simulink model "CubeQuat"  (R2016a)
settings: Solver=ode45  StartTime=0.0  StopTime=t_stop  RelTol=rel_tol
values from neighbouring files (symbols this model uses):
  adr1 = ADRblockGen(wo1,I(1,1),3)    [CubeQuat_setup.m]
  adr2 = ADRblockGen(wo2,I(2,2),3)    [CubeQuat_setup.m]    (also in WBC_setup.m = ADRblockGen(w2,m,3))
  adr3 = ADRblockGen(wo3,I(3,3),3)    [CubeQuat_setup.m]
  control_selec = 2    [CubeQuat_setup.m]
  distrej1 = 1    [CubeQuat_setup.m]
  distrej2 = 1    [CubeQuat_setup.m]
  distrej3 = 1    [CubeQuat_setup.m]
  euler_init = [0;0;0]    [CubeQuat_setup.m]
  I = diag(I_mom) + [0 I_prd(1) I_prd(2); I_prd(1) 0 I_prd(3); I_prd(2) I_prd(3) 0]    [CubeQuat_setup.m]    (also in CubeSatModel.m = reshape(I,3,3); CubeSatSfun.m = block.DialogPrm(2).Data; CubeSimSetUp.m = diag([Ixx;Iyy;Izz]); Satellite_Setup.m = diag([Ixx;Iyy;Izz]))
  in_cond_selec = 1    [CubeQuat_setup.m]
  k1 = 10    [CubeQuat_setup.m]    (also in WS_20_09_2017.mat = 5e-08; WS_25_09_2017.mat = 5e-08)
  k2 = 10    [CubeQuat_setup.m]    (also in WBC_setup.m = 5e-09; WS_20_09_2017.mat = 5e-09; WS_25_09_2017.mat = 5e-09; WS_29_09_2017.mat = 1.56433333333e-08)
  k3 = 10    [CubeQuat_setup.m]
  kd = 6e-4    (= 0.0006)    [Control_mission_def.m]    (also in CubeQuat_setup.m = 2*sqrt(I(1,1))*sqrt(kp); CubeSimSetUp.m; Example__simulaltion.m; Example_simulaltion.m)
  kp = 5e-9    (= 5e-09)    [Control_mission_def.m]    (also in CubeQuat_setup.m = 40; CubeSimSetUp.m; Example__simulaltion.m; Example_simulaltion.m)
  M = zeros(3,1)    [CubeQuat_setup.m]
  mass = 15    [CubeQuat_setup.m]    (also in CubeSimSetUp.m = 2.6; Satellite_Setup.m = 2.6; Satellite_Setup_Sun_Pointing.m = 2.6; Satellite_setup_ZenithPointing.m = 2.6)
  omega_0 = [30;30;30]*(1/sqrt(3))*(pi/180)    [CubeQuat_setup.m]
  omega_orbit = [0;-7.67/(401.1+6371);0]    [CubeQuat_setup.m]    (also in CubeSatModel.m = inputs(28:30); CubeSatSfun.m = block.DialogPrm(3).Data; CubeSimSetUp.m; Satellite_Setup.m)
  x = inputs(1:18)    [CubeSatModel.m]
  x_0 = [0,0,0,1,0,0,0]    [CubeQuat_setup.m]    (also in CubeSimSetUp.m = [wb_bi_init;qb_o_init;qb_i_init;qo_i_init;long_init;lat_init; Example__simulaltion.m = transpose([wb_bi_init,qb_i_init]); Example_simulaltion.m = transpose([wb_bi_init,qb_i_init]); Satellite_Setup.m = transpose([wb_bi_init,qb_i_init]))
undefined symbols (not defined in the file or in its folder): rotationalDynamics
libraries: cstblocks x24, aerolibtransform2 x3
settings Model: Creator=Daire  LastModifiedBy=vicubso
settings DataIOCC: LimitDataPoints=on  SaveFormat=Array
settings DebuggingCC: SolverPrmCheckMsg=warning
settings HardwareCC: ProdBitPerPointer=32  ProdLargestAtomicFloat=None  ProdIntDivRoundTo=Undefined  ProdEndianess=Unspecified  ProdWordSize=32  ProdHWDeviceType=32-bit Generic
settings ModelReferenceCC: PropagateSignalLabelsOutOfModel=off
settings ConfigComp: CovModelRefEnable=Off  CovSFcnEnable=off
settings ConfigurationSet: Description=SimMechanics 2G

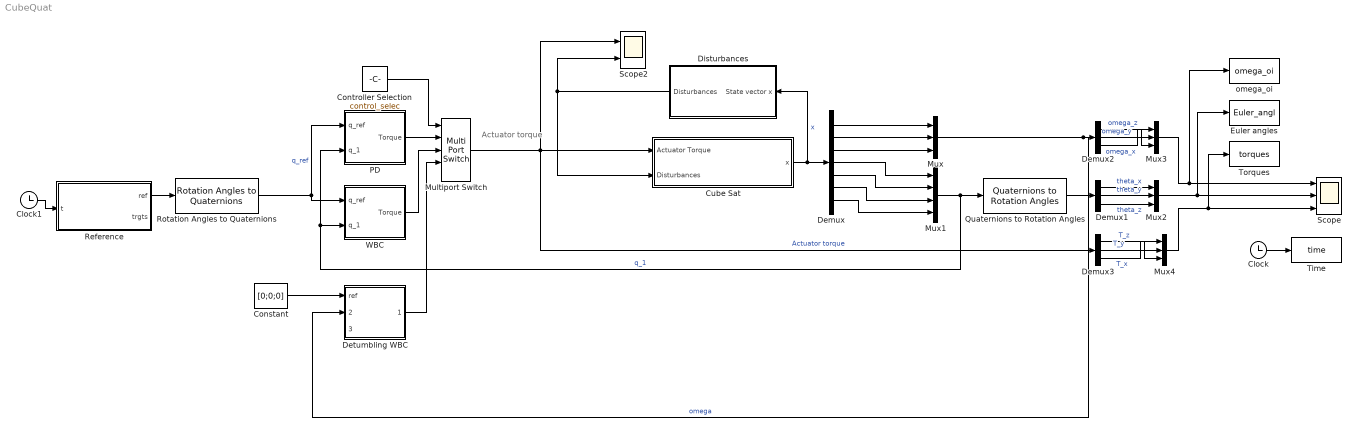
== system CubeQuat ==
  note: Actuator torque
  Clock : Clock
  Clock1 : Clock
  Constant : Constant  Value=[0;0;0]
  Controller Selection : Constant  Value=control_selec
  Cube Sat : Subsystem
  Demux : Demux  Outputs=7
  Demux1 : Demux  Outputs=3
  Demux2 : Demux  Outputs=3
  Demux3 : Demux  Outputs=3
  Detumbling WBC : Subsystem
  Disturbances : Subsystem
  Euler angles : ToWorkspace  VariableName=Euler_angl  SampleTime=-1
  Multiport Switch : MultiPortSwitch  Inputs=4
  Mux{,2..4} (4 alike) : Mux  Inputs=3
  Mux1 : Mux
  PD : Subsystem
  Quaternions to Rotation Angles : aerolibtransform2/Quaternions to Rotation Angles  rotationOrder=ZYX
  Reference : MATLAB Function  TreatAsAtomicUnit=on
  Rotation Angles to Quaternions : aerolibtransform2/Rotation Angles to Quaternions  rotationOrder=ZYX
  Scope : Scope  NumInputPorts=3
  Scope2 : Scope  NumInputPorts=2
  Time : ToWorkspace  VariableName=time  SampleTime=-1
  Torques : ToWorkspace  VariableName=torques  SampleTime=-1
  WBC : Subsystem
  omega_oi : ToWorkspace  VariableName=omega_oi  SampleTime=-1
  wires:
  Demux/1 -> Mux/1
  Demux/2 -> Mux/2
  Demux/3 -> Mux/3
  Demux/4 -> Mux1/1
  Demux/5 -> Mux1/2
  Demux/6 -> Mux1/3
  Demux/7 -> Mux1/4
  Mux1/1 -> Quaternions to Rotation Angles/1, PD/2(q_1), WBC/2(q_1)  "q_1"
  Quaternions to Rotation Angles/1 -> Demux1/1
  Rotation Angles to Quaternions/1 -> PD/1(q_ref), WBC/1(q_ref)  "q_ref"
  Demux1/1 -> Mux2/1  "theta_x"
  Demux1/2 -> Mux2/2  "theta_y"
  Demux1/3 -> Mux2/3  "theta_z"
  Mux2/1 -> Euler angles/1, Scope/2
  Mux/1 -> Detumbling WBC/2(omega), Demux2/1  "omega"
  Demux2/1 -> Mux3/3  "omega_z"
  Demux2/2 -> Mux3/2  "omega_y"
  Demux2/3 -> Mux3/1  "omega_x"
  Mux3/1 -> Scope/1, omega_oi/1
  Cube Sat/1(x) -> Disturbances/1(State vector x), Demux/1  "x"
  Multiport Switch/1 -> Scope2/1, Demux3/1, Cube Sat/1(Actuator Torque)  "Actuator torque"
  PD/1(Torque) -> Multiport Switch/2
  Mux4/1 -> Torques/1, Scope/3
  Demux3/1 -> Mux4/3  "T_z"
  Demux3/3 -> Mux4/1  "T_x"
  Demux3/2 -> Mux4/2  "T_y"
  Controller Selection/1 -> Multiport Switch/1
  Clock/1 -> Time/1
  WBC/1(Torque) -> Multiport Switch/3
  Disturbances/1(Disturbances) -> Cube Sat/2(Disturbances), Scope2/2
  Constant/1 -> Detumbling WBC/1(ref)
  Detumbling WBC/1(Torque) -> Multiport Switch/4
  Clock1/1 -> Reference/1(t)
  Reference/1(ref) -> Rotation Angles to Quaternions/1

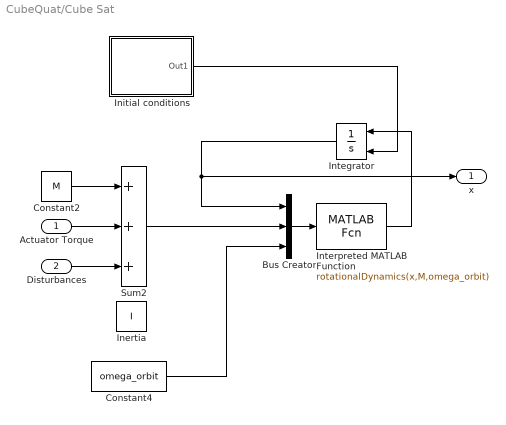
== system CubeQuat/Cube Sat ==
  Actuator Torque : Inport
  Disturbances : Inport  Port=2
  Bus Creator : BusCreator  Inputs=3
  Constant2 : Constant  Value=M
  Constant4 : Constant  Value=omega_orbit
  Inertia : Constant  Value=I
  Initial conditions : Subsystem
  Integrator : Integrator  InitialConditionSource=external
  Interpreted MATLAB Function : MATLABFcn  MATLABFcn=rotationalDynamics(x,M,omega_orbit)  OutputDimensions=1
  Sum2 : Sum  Inputs=+++
  x : Outport
  wires:
  Sum2/1 -> Bus Creator/2
  Integrator/1 -> Bus Creator/1, x/1
  Constant2/1 -> Sum2/1
  Interpreted MATLAB Function/1 -> Integrator/1
  Actuator Torque/1 -> Sum2/2
  Initial conditions/1(Out1) -> Integrator/2
  Constant4/1 -> Bus Creator/3
  Disturbances/1 -> Sum2/3
  Bus Creator/1 -> Interpreted MATLAB Function/1

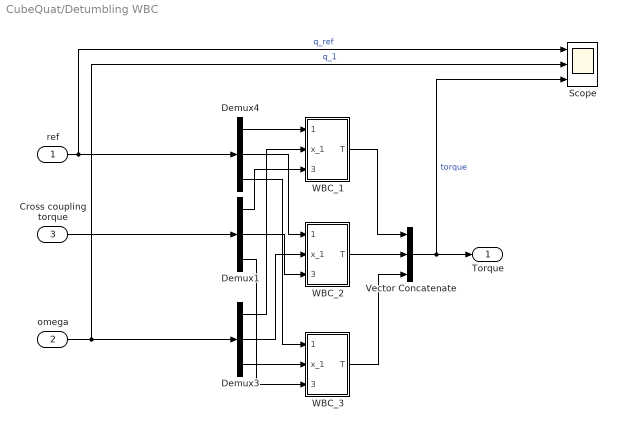
== system CubeQuat/Detumbling WBC ==
  ref : Inport
  omega : Inport  Port=2
  Cross coupling torque : Inport  Port=3
  Demux1 : Demux  Outputs=3
  Demux3 : Demux  Outputs=3
  Demux4 : Demux  Outputs=3
  Scope : Scope  NumInputPorts=3
  Vector Concatenate : Concatenate  NumInputs=3
  WBC_1 : Subsystem
  WBC_2 : Subsystem
  WBC_3 : Subsystem
  Torque : Outport
  wires:
  Demux1/3 -> WBC_3/3(Cross coupling torque)
  Demux1/2 -> WBC_2/3(Cross coupling torque)
  Demux1/1 -> WBC_1/3(Cross coupling torque)
  Cross coupling torque/1 -> Demux1/1
  WBC_1/1(T) -> Vector Concatenate/1
  Demux3/1 -> WBC_1/2(x_1)
  Demux3/2 -> WBC_2/2(x_1)
  Demux4/2 -> WBC_2/1(x_0_ref)
  ref/1 -> Demux4/1, Scope/1  "q_ref"
  WBC_3/1(T) -> Vector Concatenate/3
  Vector Concatenate/1 -> Scope/3, Torque/1  "torque"
  WBC_2/1(T) -> Vector Concatenate/2
  Demux4/3 -> WBC_3/1(x_0_ref)
  Demux4/1 -> WBC_1/1(x_0_ref)
  omega/1 -> Demux3/1, Scope/2  "q_1"
  Demux3/3 -> WBC_3/2(x_1)

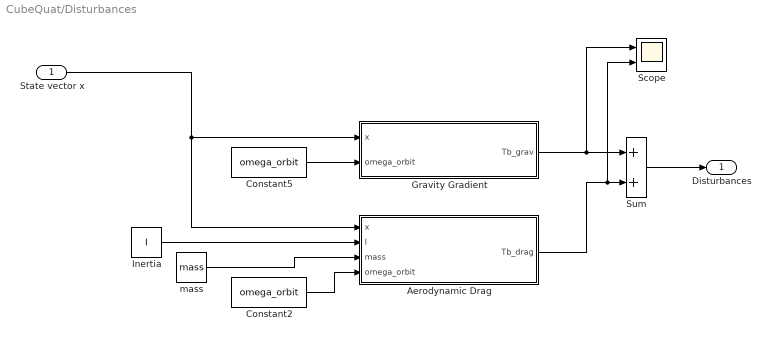
== system CubeQuat/Disturbances ==
  State vector x : Inport
  Aerodynamic Drag : MATLAB Function  TreatAsAtomicUnit=on
  Constant2 : Constant  Value=omega_orbit
  Constant5 : Constant  Value=omega_orbit
  Gravity Gradient : MATLAB Function  TreatAsAtomicUnit=on
  Inertia : Constant  Value=I
  Scope : Scope  NumInputPorts=2
  Sum : Sum
  mass : Constant  Value=mass
  Disturbances : Outport
  wires:
  Aerodynamic Drag/1(Tb_drag) -> Scope/2, Sum/2
  mass/1 -> Aerodynamic Drag/3(mass)
  Constant5/1 -> Gravity Gradient/2(omega_orbit)
  Constant2/1 -> Aerodynamic Drag/4(omega_orbit)
  Inertia/1 -> Aerodynamic Drag/2(I)
  State vector x/1 -> Gravity Gradient/1(x), Aerodynamic Drag/1(x)
  Sum/1 -> Disturbances/1
  Gravity Gradient/1(Tb_grav) -> Scope/1, Sum/1

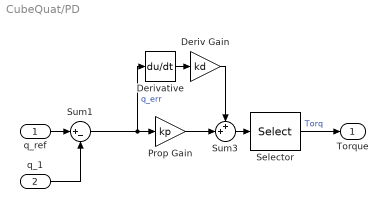
== system CubeQuat/PD ==
  q_ref : Inport
  q_1 : Inport  Port=2
  Deriv Gain : Gain  Gain=kd
  Derivative : Derivative
  Prop Gain : Gain  Gain=kp
  Selector : Selector  InputPortWidth=4  IndexOptions=Index vector (dialog)  Indices=[2,3,4]  OutputSizes=1
  Sum1 : Sum  Inputs=|+-
  Sum3 : Sum  Inputs=++|
  Torque : Outport
  wires:
  Selector/1 -> Torque/1  "Torq"
  Deriv Gain/1 -> Sum3/1
  Derivative/1 -> Deriv Gain/1
  Prop Gain/1 -> Sum3/2
  Sum1/1 -> Prop Gain/1, Derivative/1  "q_err"
  q_1/1 -> Sum1/2
  q_ref/1 -> Sum1/1
  Sum3/1 -> Selector/1

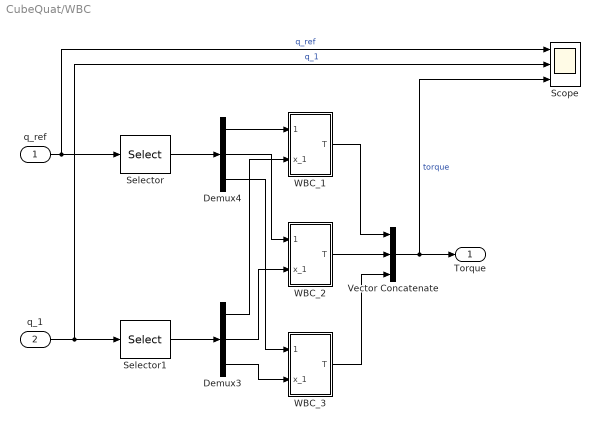
== system CubeQuat/WBC ==
  q_ref : Inport
  q_1 : Inport  Port=2
  Demux3 : Demux  Outputs=3
  Demux4 : Demux  Outputs=3
  Scope : Scope  NumInputPorts=3
  Selector : Selector  InputPortWidth=4  IndexOptions=Index vector (dialog)  Indices=[2,3,4]  OutputSizes=1
  Selector1 : Selector  InputPortWidth=4  IndexOptions=Index vector (dialog)  Indices=[2,3,4]  OutputSizes=1
  Vector Concatenate : Concatenate  NumInputs=3
  WBC_1 : Subsystem
  WBC_2 : Subsystem
  WBC_3 : Subsystem
  Torque : Outport
  wires:
  Demux3/3 -> WBC_3/2(x_1)
  q_1/1 -> Scope/2, Selector1/1  "q_1"
  Demux4/1 -> WBC_1/1(x_0_ref)
  Demux4/3 -> WBC_3/1(x_0_ref)
  WBC_2/1(T) -> Vector Concatenate/2
  Vector Concatenate/1 -> Torque/1, Scope/3  "torque"
  WBC_3/1(T) -> Vector Concatenate/3
  q_ref/1 -> Selector/1, Scope/1  "q_ref"
  Selector/1 -> Demux4/1
  Demux4/2 -> WBC_2/1(x_0_ref)
  Selector1/1 -> Demux3/1
  Demux3/2 -> WBC_2/2(x_1)
  Demux3/1 -> WBC_1/2(x_1)
  WBC_1/1(T) -> Vector Concatenate/1

== system CubeQuat/Cube Sat/Initial conditions ==
  Initial Cond. Selector : Constant  Value=in_cond_selec
  Initial Conditions : Constant  Value=x_0
  Initial Conditions1 : Constant  Value=omega_0
  Initial Conditions2 : Constant  Value=euler_init
  Mux : Mux  Inputs=2
  Rotation Angles to Quaternions : aerolibtransform2/Rotation Angles to Quaternions  rotationOrder=ZYX
  Switch : Switch  Criteria=u2 ~= 0
  Out1 : Outport
  wires:
  Initial Conditions/1 -> Switch/1
  Rotation Angles to Quaternions/1 -> Mux/2
  Switch/1 -> Out1/1
  Mux/1 -> Switch/3
  Initial Conditions1/1 -> Mux/1
  Initial Conditions2/1 -> Rotation Angles to Quaternions/1
  Initial Cond. Selector/1 -> Switch/2

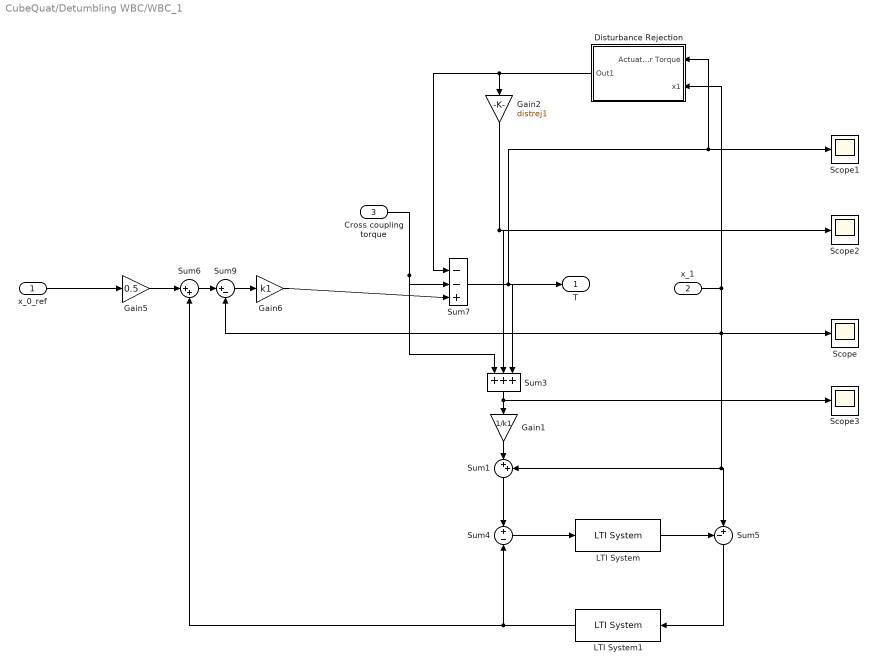
== system CubeQuat/Detumbling WBC/WBC_1 ==
  x_0_ref : Inport
  x_1 : Inport  Port=2
  Cross coupling torque : Inport  Port=3
  Disturbance Rejection : Subsystem
  Gain1 : Gain  Gain=1/k1
  Gain2 : Gain  Gain=distrej1
  Gain5 : Gain  Gain=0.5
  Gain6 : Gain  Gain=k1
  LTI System : cstblocks/LTI System  sys=G1  IC=[]
  LTI System1 : cstblocks/LTI System  sys=G1  IC=[]
  Scope{,1..3} (4 alike) : Scope
  Sum1 : Sum  Inputs=|++
  Sum3 : Sum  Inputs=+++|
  Sum4 : Sum  Inputs=+|-
  Sum5 : Sum  Inputs=-+|
  Sum6 : Sum  Inputs=|++
  Sum7 : Sum  Inputs=--+|
  Sum9 : Sum  Inputs=|+-
  T : Outport
  wires:
  Cross coupling torque/1 -> Sum7/2, Sum3/1
  Disturbance Rejection/1(Out1) -> Gain2/1, Sum7/1
  x_1/1 -> Disturbance Rejection/2(x1), Sum9/2, Scope/1, Sum5/2, Sum1/2
  Gain1/1 -> Sum1/1
  LTI System1/1 -> Sum6/2, Sum4/2
  Gain2/1 -> Scope2/1, Sum3/2
  Gain6/1 -> Sum7/3
  Sum3/1 -> Gain1/1, Scope3/1
  Sum6/1 -> Sum9/1
  x_0_ref/1 -> Gain5/1
  Sum9/1 -> Gain6/1
  Sum7/1 -> T/1, Sum3/3, Disturbance Rejection/1(Actuator Torque), Scope1/1
  Gain5/1 -> Sum6/1
  Sum4/1 -> LTI System/1
  LTI System/1 -> Sum5/1
  Sum5/1 -> LTI System1/1
  Sum1/1 -> Sum4/1

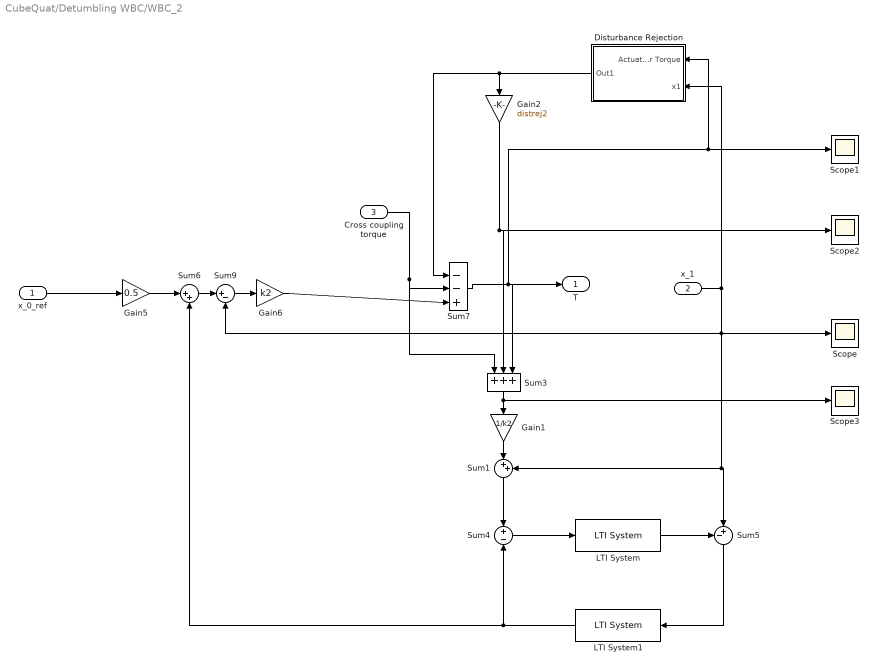
== system CubeQuat/Detumbling WBC/WBC_2 ==
  x_0_ref : Inport
  x_1 : Inport  Port=2
  Cross coupling torque : Inport  Port=3
  Disturbance Rejection : Subsystem
  Gain1 : Gain  Gain=1/k2
  Gain2 : Gain  Gain=distrej2
  Gain5 : Gain  Gain=0.5
  Gain6 : Gain  Gain=k2
  LTI System : cstblocks/LTI System  sys=G2  IC=[]
  LTI System1 : cstblocks/LTI System  sys=G2  IC=[]
  Scope{,1..3} (4 alike) : Scope
  Sum1 : Sum  Inputs=|++
  Sum3 : Sum  Inputs=+++|
  Sum4 : Sum  Inputs=+|-
  Sum5 : Sum  Inputs=-+|
  Sum6 : Sum  Inputs=|++
  Sum7 : Sum  Inputs=--+|
  Sum9 : Sum  Inputs=|+-
  T : Outport
  wires:
  Cross coupling torque/1 -> Sum3/1, Sum7/2
  Disturbance Rejection/1(Out1) -> Gain2/1, Sum7/1
  x_1/1 -> Disturbance Rejection/2(x1), Sum9/2, Scope/1, Sum5/2, Sum1/2
  Gain1/1 -> Sum1/1
  LTI System1/1 -> Sum6/2, Sum4/2
  Gain2/1 -> Scope2/1, Sum3/2
  Gain6/1 -> Sum7/3
  Sum3/1 -> Gain1/1, Scope3/1
  Sum6/1 -> Sum9/1
  x_0_ref/1 -> Gain5/1
  Sum9/1 -> Gain6/1
  Sum7/1 -> T/1, Sum3/3, Disturbance Rejection/1(Actuator Torque), Scope1/1
  Gain5/1 -> Sum6/1
  Sum4/1 -> LTI System/1
  LTI System/1 -> Sum5/1
  Sum5/1 -> LTI System1/1
  Sum1/1 -> Sum4/1

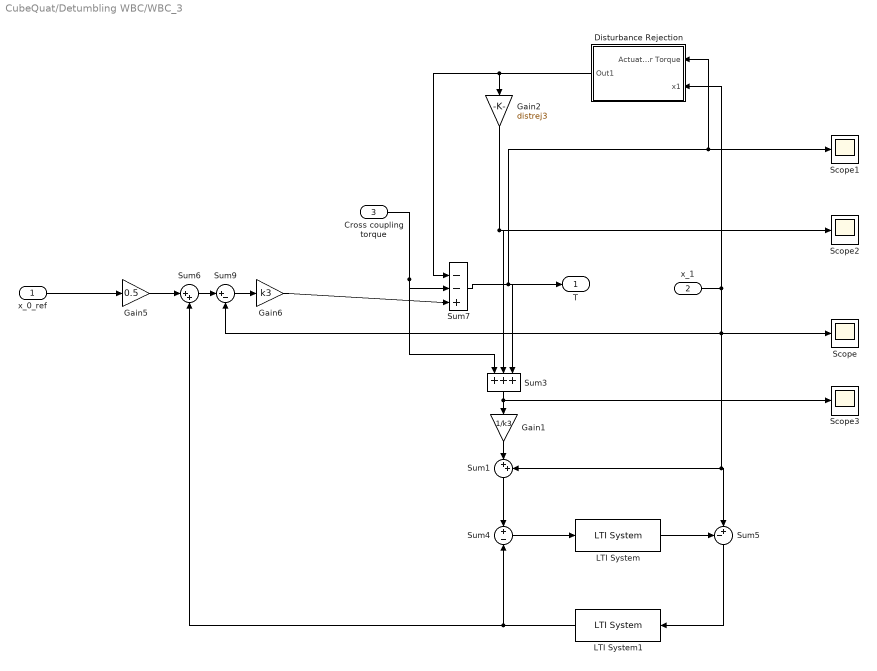
== system CubeQuat/Detumbling WBC/WBC_3 ==
  x_0_ref : Inport
  x_1 : Inport  Port=2
  Cross coupling torque : Inport  Port=3
  Disturbance Rejection : Subsystem
  Gain1 : Gain  Gain=1/k3
  Gain2 : Gain  Gain=distrej3
  Gain5 : Gain  Gain=0.5
  Gain6 : Gain  Gain=k3
  LTI System : cstblocks/LTI System  sys=G3  IC=[]
  LTI System1 : cstblocks/LTI System  sys=G3  IC=[]
  Scope{,1..3} (4 alike) : Scope
  Sum1 : Sum  Inputs=|++
  Sum3 : Sum  Inputs=+++|
  Sum4 : Sum  Inputs=+|-
  Sum5 : Sum  Inputs=-+|
  Sum6 : Sum  Inputs=|++
  Sum7 : Sum  Inputs=--+|
  Sum9 : Sum  Inputs=|+-
  T : Outport
  wires:
  Cross coupling torque/1 -> Sum3/1, Sum7/2
  Disturbance Rejection/1(Out1) -> Gain2/1, Sum7/1
  x_1/1 -> Disturbance Rejection/2(x1), Sum9/2, Scope/1, Sum5/2, Sum1/2
  Gain1/1 -> Sum1/1
  LTI System1/1 -> Sum6/2, Sum4/2
  Gain2/1 -> Scope2/1, Sum3/2
  Gain6/1 -> Sum7/3
  Sum3/1 -> Gain1/1, Scope3/1
  Sum6/1 -> Sum9/1
  x_0_ref/1 -> Gain5/1
  Sum9/1 -> Gain6/1
  Sum7/1 -> T/1, Sum3/3, Disturbance Rejection/1(Actuator Torque), Scope1/1
  Gain5/1 -> Sum6/1
  Sum4/1 -> LTI System/1
  LTI System/1 -> Sum5/1
  Sum5/1 -> LTI System1/1
  Sum1/1 -> Sum4/1

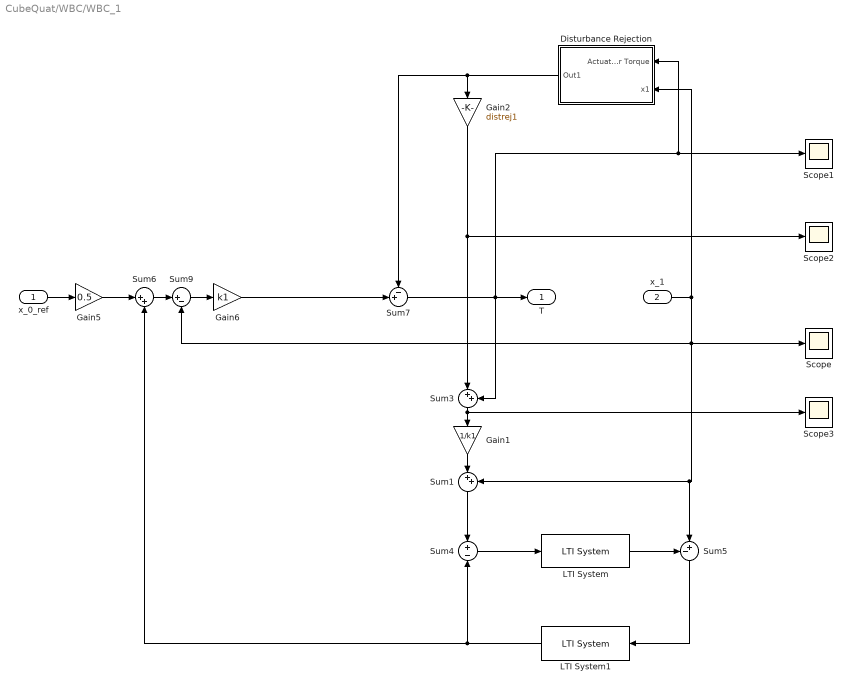
== system CubeQuat/WBC/WBC_1 ==
  x_0_ref : Inport
  x_1 : Inport  Port=2
  Disturbance Rejection : Subsystem
  Gain1 : Gain  Gain=1/k1
  Gain2 : Gain  Gain=distrej1
  Gain5 : Gain  Gain=0.5
  Gain6 : Gain  Gain=k1
  LTI System : cstblocks/LTI System  sys=G1  IC=[]
  LTI System1 : cstblocks/LTI System  sys=G1  IC=[]
  Scope{,1..3} (4 alike) : Scope
  Sum1 : Sum  Inputs=|++
  Sum3 : Sum  Inputs=|++
  Sum4 : Sum  Inputs=+|-
  Sum5 : Sum  Inputs=-+|
  Sum6 : Sum  Inputs=|++
  Sum7 : Sum  Inputs=-+|
  Sum9 : Sum  Inputs=|+-
  T : Outport
  wires:
  Sum1/1 -> Sum4/1
  Sum5/1 -> LTI System1/1
  LTI System/1 -> Sum5/1
  Sum4/1 -> LTI System/1
  Gain5/1 -> Sum6/1
  Sum7/1 -> Scope1/1, Disturbance Rejection/1(Actuator Torque), Sum3/2, T/1
  Sum9/1 -> Gain6/1
  x_0_ref/1 -> Gain5/1
  Sum6/1 -> Sum9/1
  Sum3/1 -> Scope3/1, Gain1/1
  Gain6/1 -> Sum7/2
  Gain2/1 -> Sum3/1, Scope2/1
  LTI System1/1 -> Sum4/2, Sum6/2
  Gain1/1 -> Sum1/1
  x_1/1 -> Sum1/2, Sum5/2, Scope/1, Sum9/2, Disturbance Rejection/2(x1)
  Disturbance Rejection/1(Out1) -> Sum7/1, Gain2/1

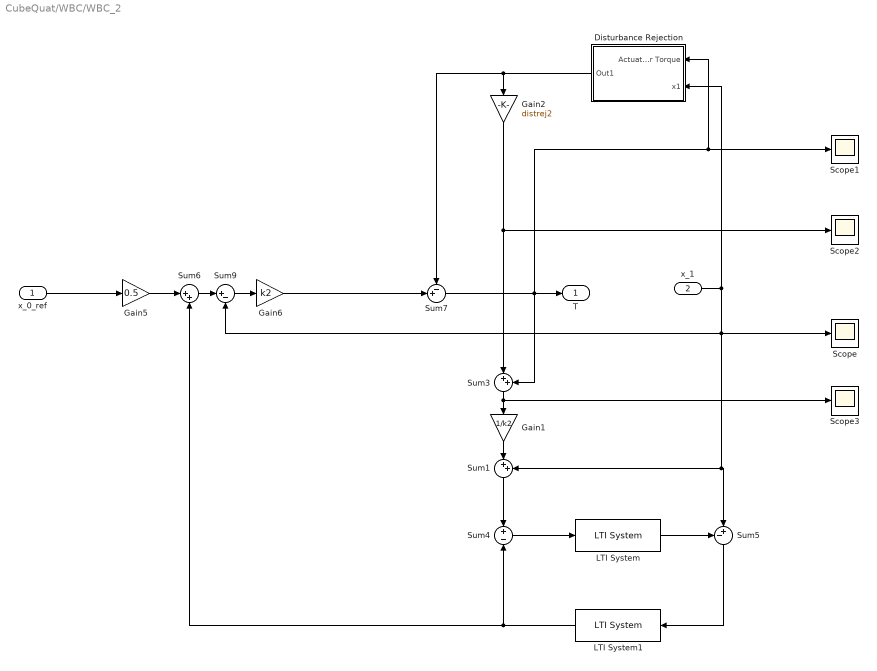
== system CubeQuat/WBC/WBC_2 ==
  x_0_ref : Inport
  x_1 : Inport  Port=2
  Disturbance Rejection : Subsystem
  Gain1 : Gain  Gain=1/k2
  Gain2 : Gain  Gain=distrej2
  Gain5 : Gain  Gain=0.5
  Gain6 : Gain  Gain=k2
  LTI System : cstblocks/LTI System  sys=G2  IC=[]
  LTI System1 : cstblocks/LTI System  sys=G2  IC=[]
  Scope{,1..3} (4 alike) : Scope
  Sum1 : Sum  Inputs=|++
  Sum3 : Sum  Inputs=|++
  Sum4 : Sum  Inputs=+|-
  Sum5 : Sum  Inputs=-+|
  Sum6 : Sum  Inputs=|++
  Sum7 : Sum  Inputs=-+|
  Sum9 : Sum  Inputs=|+-
  T : Outport
  wires:
  Sum1/1 -> Sum4/1
  Sum5/1 -> LTI System1/1
  LTI System/1 -> Sum5/1
  Sum4/1 -> LTI System/1
  Gain5/1 -> Sum6/1
  Sum7/1 -> T/1, Sum3/2, Scope1/1, Disturbance Rejection/1(Actuator Torque)
  Sum9/1 -> Gain6/1
  x_0_ref/1 -> Gain5/1
  Sum6/1 -> Sum9/1
  Sum3/1 -> Scope3/1, Gain1/1
  Gain6/1 -> Sum7/2
  Gain2/1 -> Sum3/1, Scope2/1
  LTI System1/1 -> Sum4/2, Sum6/2
  Gain1/1 -> Sum1/1
  x_1/1 -> Sum1/2, Sum5/2, Scope/1, Sum9/2, Disturbance Rejection/2(x1)
  Disturbance Rejection/1(Out1) -> Sum7/1, Gain2/1

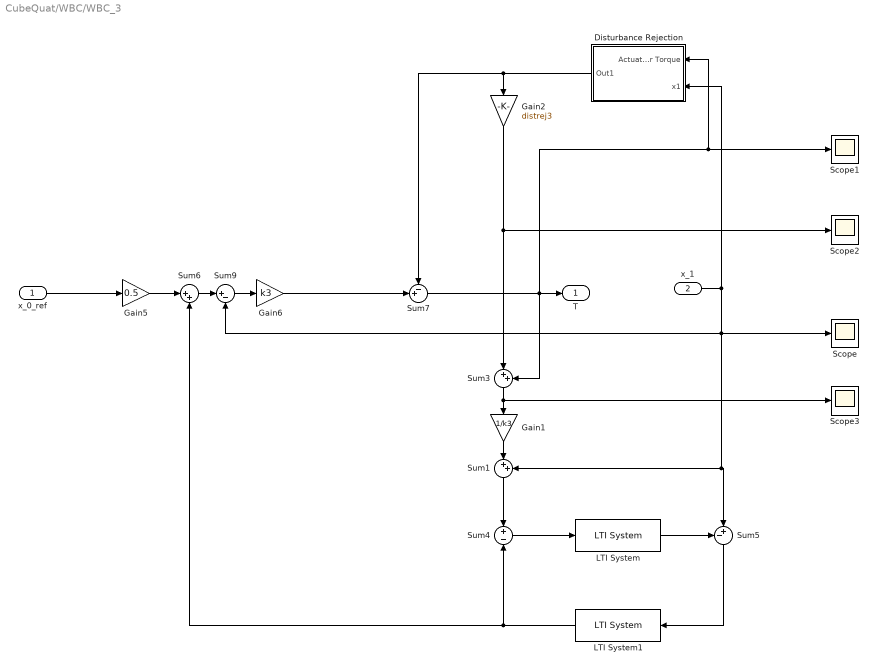
== system CubeQuat/WBC/WBC_3 ==
  x_0_ref : Inport
  x_1 : Inport  Port=2
  Disturbance Rejection : Subsystem
  Gain1 : Gain  Gain=1/k3
  Gain2 : Gain  Gain=distrej3
  Gain5 : Gain  Gain=0.5
  Gain6 : Gain  Gain=k3
  LTI System : cstblocks/LTI System  sys=G3  IC=[]
  LTI System1 : cstblocks/LTI System  sys=G3  IC=[]
  Scope{,1..3} (4 alike) : Scope
  Sum1 : Sum  Inputs=|++
  Sum3 : Sum  Inputs=|++
  Sum4 : Sum  Inputs=+|-
  Sum5 : Sum  Inputs=-+|
  Sum6 : Sum  Inputs=|++
  Sum7 : Sum  Inputs=-+|
  Sum9 : Sum  Inputs=|+-
  T : Outport
  wires:
  Sum1/1 -> Sum4/1
  Sum5/1 -> LTI System1/1
  LTI System/1 -> Sum5/1
  Sum4/1 -> LTI System/1
  Gain5/1 -> Sum6/1
  Sum7/1 -> Sum3/2, Scope1/1, Disturbance Rejection/1(Actuator Torque), T/1
  Sum9/1 -> Gain6/1
  x_0_ref/1 -> Gain5/1
  Sum6/1 -> Sum9/1
  Sum3/1 -> Scope3/1, Gain1/1
  Gain6/1 -> Sum7/2
  Gain2/1 -> Sum3/1, Scope2/1
  LTI System1/1 -> Sum4/2, Sum6/2
  Gain1/1 -> Sum1/1
  x_1/1 -> Sum1/2, Sum5/2, Scope/1, Sum9/2, Disturbance Rejection/2(x1)
  Disturbance Rejection/1(Out1) -> Sum7/1, Gain2/1

== system CubeQuat/Detumbling WBC/WBC_1/Disturbance Rejection ==
  note: Subsystem
  Actuator Torque : Inport
  x1 : Inport  Port=2
  LTI System2 : cstblocks/LTI System  sys=adr1(1)  IC=[]
  LTI System3 : cstblocks/LTI System  sys=adr1(2)  IC=[]
  Sum2 : Sum  Inputs=|++
  Out1 : Outport
  wires:
  LTI System3/1 -> Sum2/2
  Actuator Torque/1 -> LTI System3/1
  x1/1 -> LTI System2/1
  LTI System2/1 -> Sum2/1
  Sum2/1 -> Out1/1

== system CubeQuat/Detumbling WBC/WBC_2/Disturbance Rejection ==
  note: Subsystem
  Actuator Torque : Inport
  x1 : Inport  Port=2
  LTI System2 : cstblocks/LTI System  sys=adr2(1)  IC=[]
  LTI System3 : cstblocks/LTI System  sys=adr2(2)  IC=[]
  Sum2 : Sum  Inputs=|++
  Out1 : Outport
  wires:
  LTI System3/1 -> Sum2/2
  Actuator Torque/1 -> LTI System3/1
  x1/1 -> LTI System2/1
  LTI System2/1 -> Sum2/1
  Sum2/1 -> Out1/1

== system CubeQuat/Detumbling WBC/WBC_3/Disturbance Rejection ==
  note: Subsystem
  Actuator Torque : Inport
  x1 : Inport  Port=2
  LTI System2 : cstblocks/LTI System  sys=adr3(1)  IC=[]
  LTI System3 : cstblocks/LTI System  sys=adr3(2)  IC=[]
  Sum2 : Sum  Inputs=|++
  Out1 : Outport
  wires:
  LTI System3/1 -> Sum2/2
  Actuator Torque/1 -> LTI System3/1
  x1/1 -> LTI System2/1
  LTI System2/1 -> Sum2/1
  Sum2/1 -> Out1/1

== system CubeQuat/WBC/WBC_1/Disturbance Rejection ==
  note: Subsystem
  Actuator Torque : Inport
  x1 : Inport  Port=2
  LTI System2 : cstblocks/LTI System  sys=adr1(1)  IC=[]
  LTI System3 : cstblocks/LTI System  sys=adr1(2)  IC=[]
  Sum2 : Sum  Inputs=|++
  Out1 : Outport
  wires:
  Sum2/1 -> Out1/1
  LTI System2/1 -> Sum2/1
  x1/1 -> LTI System2/1
  Actuator Torque/1 -> LTI System3/1
  LTI System3/1 -> Sum2/2

== system CubeQuat/WBC/WBC_2/Disturbance Rejection ==
  note: Subsystem
  Actuator Torque : Inport
  x1 : Inport  Port=2
  LTI System2 : cstblocks/LTI System  sys=adr2(1)  IC=[]
  LTI System3 : cstblocks/LTI System  sys=adr2(2)  IC=[]
  Sum2 : Sum  Inputs=|++
  Out1 : Outport
  wires:
  Sum2/1 -> Out1/1
  LTI System2/1 -> Sum2/1
  x1/1 -> LTI System2/1
  Actuator Torque/1 -> LTI System3/1
  LTI System3/1 -> Sum2/2

== system CubeQuat/WBC/WBC_3/Disturbance Rejection ==
  note: Subsystem
  Actuator Torque : Inport
  x1 : Inport  Port=2
  LTI System2 : cstblocks/LTI System  sys=adr3(1)  IC=[]
  LTI System3 : cstblocks/LTI System  sys=adr3(2)  IC=[]
  Sum2 : Sum  Inputs=|++
  Out1 : Outport
  wires:
  Sum2/1 -> Out1/1
  LTI System2/1 -> Sum2/1
  x1/1 -> LTI System2/1
  Actuator Torque/1 -> LTI System3/1
  LTI System3/1 -> Sum2/2

== matlab function CubeQuat/Disturbances/Gravity Gradient ==
  data: x input; omega_orbit input; Tb_grav output
function Tb_grav = gravGradient(x,omega_orbit)

%Computes the gravity gradient torque. 
%According to 'Attitude Control System of a Double CubeSat - Gaute Brathen'

%Inputs:

% - x: state vector, from which the quaternion will be extracted 
%       x = [omega(3x1);q(4x1)]
%       q = [eta;epsilon] = [x(4),x(5:7)]
% - omega_orbit: orbital angular velocity wrt inertial frame, expressed in
%   orbital frame. 
%   eg. for an polar orbit, it would take the form [0, -w_io, o]

%Extract the quaternion from the state vector
q=x(4:7);
n=q(1);
eps=q(2:4);

%Skew-simmetric associated with the quaternion's vector part
S = SkewSym(eps);

%Rotation matrices between orbit and body frame
Ro_b = eye(3) + (2*n*S) + (2*(S^2)); %Transforms from the body frame to the orbital frame
Rb_o = transpose(Ro_b); %Transforms from the orbital frame to the body frame

c_3=Rb_o(:,3); %3rd Column

Tb_grav=3*(omega_orbit(2)^2)*SkewSym(c_3)*eye(3)*c_3;

return;

== matlab function CubeQuat/Disturbances/Aerodynamic Drag ==
  data: x input; I input; Tb_drag output; mass input; omega_orbit input
function Tb_drag = aeroDrag(x,I,mass,omega_orbit)

%Computes the aerodynamic drag. 
%According to 'Attitude Control System of a Double CubeSat - Gaute Brathen
% sec 3.6.2

%Inputs:

% - x: state vector, from which the quaternion will be extracted 
%       x = [omega(3x1);q(4x1)]
%       q = [eta;epsilon] = [x(4),x(5:7)]
% - omega_orbit: orbital angular velocity wrt inertial frame, expressed in
%   orbital frame. 
%   eg. for an polar orbit, it would take the form [0, -w_io, o]
% - Data = [rho_a, A_p, 

%       - rho_a: atmospheric density (Kg/m^3)
%       - A_p: aerodynamic area. Set as constant, but could be
%        defined as a function of attitude.
%       - V_o_b: Unity vector of the local atmosphere velocity vector.
%        For convenience, it is usually expresed in terms of the orbital
%        frame (V_o_r), because it is parallel to the x plane; so
%        (as the torque output is expresed i.t.o. the body frame), we'll
%        need to transform it (V_b_r) using the rotation matrix Rb_o
%       - vel: magnitude of the local atmosfhere velocity
%       "Harcoded" as orbital velocity x radius
%       - J: Inertia tensor with origin the center of pressure, calculated
%       from Steiner's Theorem

%Extract the quaternion and omega from the state vector
omega = x(1:3);
q=x(4:7);
n=q(1);
eps=q(2:4);

S = SkewSym(eps); %Squew-Sym matrix associated with vector part of quaternion

%Rotation matrices between orbit and body frame
Ro_b = eye(3) + (2*n*S) + (2*(S^2)); %Transforms from the body frame to the orbital frame
Rb_o = transpose(Ro_b); %Transforms from the orbital frame to the body frame

omega_b_ob=omega-(Rb_o*omega_orbit);

rho_a = 4.89e-13; %Atmospheric density at LEO 
c_p = 0.02*[1;1;1]; %(!!!) HARDCODE Vector C.O.Mass - C.O.Pressure i.t.o. body frame
c_pSk = SkewSym(c_p); % its Skew-Sym matrix
V_o_r = [-1;0;0]; % Unity vector in the direction of the 
%                        local atmospheric velocity i.t.o. orbital frame
V_b_r = Rb_o * V_o_r; % ... in terms of body frame
VrSk = SkewSym(V_b_r); % its Skew-Sym matrix
vel = 7.664e3; %(!!!) HARDCODE magnitude of the local atmosfhere velocity
a = c_p(1)^2; b = c_p(2)^2; c = c_p(3)^2;
J = I + mass * [b+c c b; c a+c a; b a a+b]; %Inertia with origin the center of pressure. Steiner theorem
A_d = 0.2*0.1*sqrt(2); %(!!!) HARDCODE Aerodynamic area. Wrost case scenario

Tb_drag = rho_a * vel * (vel*A_d*c_pSk*V_b_r - (I + VrSk*J) * omega_b_ob);

return;

== matlab function CubeQuat/Reference ==
  data: t input; ref output; trgts output
function [ref,trgts]  = fcn(t)

%Define references r1 r2 r3 as a function of time. 

%Steps of amplitude A1 A2 A2 (deg) , at times T1 T2 T3 (sec)

T1 = 1;
T2 = 1.5;
T3 = 2;
A1 = 0.3 * (180/pi);
A2 = 0.5 * (180/pi);
A3 = 0.7 * (180/pi);

r1 = 0; r2 = 0; r3 = 0;

if t > T1; r1 = A1; end
if t > T2; r2 = A2; end
if t > T3; r3 = A3; end


trgts = [T1,T2,T3];
ref = [r1,r2,r3];

return;
